simulink model "giveathought"  (R2018a)
settings: Solver=VariableStepAuto  StartTime=0.0  StopTime=100  RelTol=1e-3
settings Model: Creator=Li Gen  LastModifiedBy=Li Gen

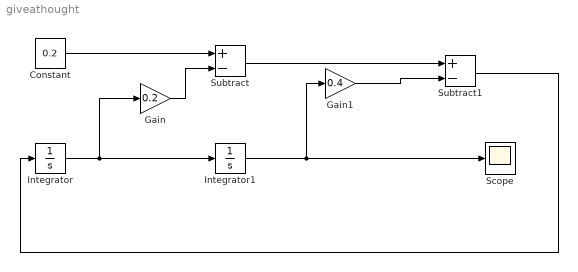
== system giveathought ==
  Constant : Constant  Value=0.2
  Gain : Gain  Gain=0.2
  Gain1 : Gain  Gain=0.4
  Integrator : Integrator
  Integrator1 : Integrator
  Scope : Scope
  Subtract : Sum  Inputs=+-
  Subtract1 : Sum  Inputs=+-
  wires:
  Integrator/1 -> Gain/1, Integrator1/1
  Constant/1 -> Subtract/1
  Integrator1/1 -> Gain1/1, Scope/1
  Gain/1 -> Subtract/2
  Gain1/1 -> Subtract1/2
  Subtract/1 -> Subtract1/1
  Subtract1/1 -> Integrator/1
